simulink model "crazyflie_stu"  (R2021b)
settings: Solver=FixedStepDiscrete  StartTime=0.0  StopTime=160  FixedStep=0.001  RelTol=1e-3
undefined symbols (not defined in the file or in its folder): DiscIntNeverNeededParam
settings Model: PauseTimes=7  Creator=Zrean  LastModifiedBy=felix
settings SolverCC: AlgebraicLoopSolver=TrustRegion
settings DataIOCC: ReturnWorkspaceOutputs=off
settings OptimizationCC: DefaultParameterBehavior=Inlined  UseDivisionForNetSlopeComputation=on  UseFloatMulNetSlope=on  UseSpecifiedMinMax=on  InlineInvariantSignals=on  PassReuseOutputArgsAs=Individual arguments  ZeroExternalMemoryAtStartup=off  ZeroInternalMemoryAtStartup=off  NoFixptDivByZeroProtection=on  EfficientFloat2IntCast=on  LifeSpan=1  EfficientTunableParamExpr=on
settings DebuggingCC: AlgebraicLoopMsg=error  ParameterTunabilityLossMsg=error  SFMachineParentedDataDiag=warning  ArithmeticOperatorsInVariantConditions=warning
settings HardwareCC: ProdBitPerPointer=32  ProdBitPerSizeT=32  ProdBitPerPtrDiffT=32  ProdLargestAtomicInteger=Long  ProdLargestAtomicFloat=Double  ProdWordSize=32  ProdHWDeviceType=ARM Compatible->ARM Cortex
settings SFSimCC: SimUseLocalCustomCode=off  MATLABDynamicMemAlloc=off  CustomCodeUndefinedFunction=UseInterfaceOnly
settings RTWCC: Description=Embedded Coder  SystemTargetFile=ert.tlc  GenCodeOnly=on  TemplateMakefile=ert_default_tmf  GenerateReport=on  RTWUseLocalCustomCode=off  BuildConfiguration=Faster Runs  IncludeHyperlinkInReport=on  LaunchReport=on  GenerateTraceInfo=on  GenerateTraceReport=on  GenerateTraceReportSl=on  GenerateTraceReportSf=on  GenerateTraceReportEml=on  GenerateCodeMetricsReport=on
settings CodeAppCC: ForceParamTrailComments=on  IgnoreCustomStorageClasses=off  OperatorAnnotations=on  SimulinkDataObjDesc=on  SFDataObjDesc=on  MATLABFcnDesc=on  InsertBlockDesc=on  StateflowObjectComments=on  MATLABSourceComments=on
settings ERTTargetCC: TargetLangStandard=C99 (ISO)  MultiwordLength=2048  CombineSignalStateStructs=on  SuppressErrorStatus=on  SupportAbsoluteTime=off  SupportNonFinite=off  SupportComplex=off  InlinedParameterPlacement=NonHierarchical  ERTCustomFileTemplate=crazyflie_wrapper.tlc  ERTFilePackagingFormat=CompactWithDataFile
settings SimscapeCC: SimscapeNormalizeSystem=off

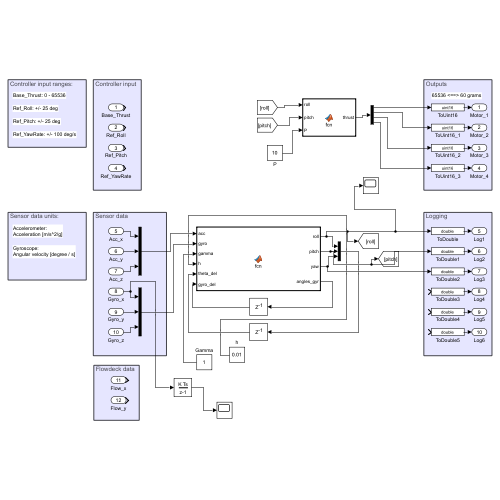
[thumbnail: Simulink's stored preview of the top-level diagram]
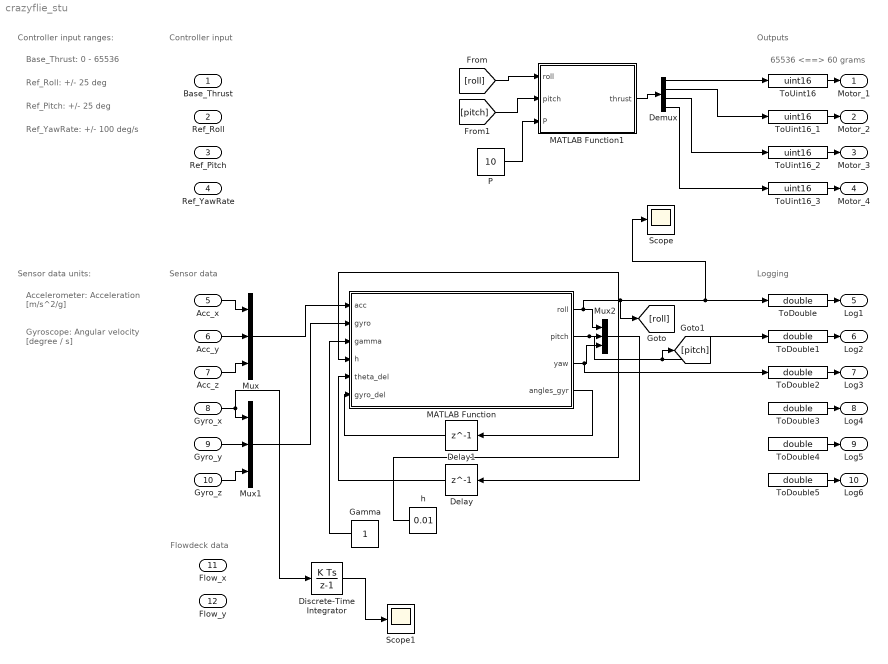
== system crazyflie_stu ==
  note: 65536 <==> 60 grams
  note: Logging
  note: Outputs
  note: Sensor data
  note: Controller input
  note: Ref_Roll: +/- 25 deg
  note: Base_Thrust: 0 - 65536
  note: Ref_Pitch: +/- 25 deg
  note: Ref_YawRate: +/- 100 deg/s
  note: Controller input ranges:
  note: Gyroscope:
      | Angular velocity [degree / s]
  note: Accelerometer:
      | Acceleration [m/s^2/g]
  note: Sensor data units:
  note: Flowdeck data
  Base_Thrust : Inport  OutDataTypeStr=double
  Ref_Roll : Inport  Port=2  OutDataTypeStr=double
  Ref_Pitch : Inport  Port=3  OutDataTypeStr=double
  Ref_YawRate : Inport  Port=4  OutDataTypeStr=double
  Acc_x : Inport  Port=5  OutDataTypeStr=double  PortDimensions=1
  Acc_y : Inport  Port=6  OutDataTypeStr=double  PortDimensions=1
  Acc_z : Inport  Port=7  OutDataTypeStr=double  PortDimensions=1
  Gyro_x : Inport  Port=8  OutDataTypeStr=double  PortDimensions=1
  Gyro_y : Inport  Port=9  OutDataTypeStr=double  PortDimensions=1
  Gyro_z : Inport  Port=10  OutDataTypeStr=double  PortDimensions=1
  Flow_x : Inport  Port=11  OutDataTypeStr=int16  PortDimensions=1
  Flow_y : Inport  Port=12  OutDataTypeStr=int16  PortDimensions=1
  Delay : Delay  DelayLength=1
  Delay1 : Delay  DelayLength=1
  Demux : Demux
  Discrete-Time Integrator : DiscreteIntegrator  SampleTime=-1  ICPrevOutput=DiscIntNeverNeededParam  ICPrevScaledInput=DiscIntNeverNeededParam
  Gamma : Constant
  MATLAB Function : MATLAB Function  TreatAsAtomicUnit=on
  MATLAB Function1 : MATLAB Function  TreatAsAtomicUnit=on
  Mux : Mux  Inputs=3
  Mux1 : Mux  Inputs=3
  Mux2 : Mux  Inputs=3
  P : Constant  Value=10
  Scope : Scope
  Scope1 : Scope
  ToDouble{,1..5} (6 alike) : DataTypeConversion  OutDataTypeStr=double  SaturateOnIntegerOverflow=on
  ToUint16 : DataTypeConversion  OutDataTypeStr=uint16  SaturateOnIntegerOverflow=on
  ToUint16_1 : DataTypeConversion  OutDataTypeStr=uint16  SaturateOnIntegerOverflow=on
  ToUint16_2 : DataTypeConversion  OutDataTypeStr=uint16  SaturateOnIntegerOverflow=on
  ToUint16_3 : DataTypeConversion  OutDataTypeStr=uint16  SaturateOnIntegerOverflow=on
  h : Constant  Value=0.01
  Motor_1 : Outport  OutDataTypeStr=uint16  VectorParamsAs1DForOutWhenUnconnected=off  LockScale=on
  Motor_2 : Outport  Port=2  OutDataTypeStr=uint16  VectorParamsAs1DForOutWhenUnconnected=off  LockScale=on
  Motor_3 : Outport  Port=3  OutDataTypeStr=uint16  VectorParamsAs1DForOutWhenUnconnected=off  LockScale=on
  Motor_4 : Outport  Port=4  OutDataTypeStr=uint16  VectorParamsAs1DForOutWhenUnconnected=off  LockScale=on
  Log1 : Outport  Port=5  OutDataTypeStr=double  VectorParamsAs1DForOutWhenUnconnected=off
  Log2 : Outport  Port=6  OutDataTypeStr=double  VectorParamsAs1DForOutWhenUnconnected=off
  Log3 : Outport  Port=7  OutDataTypeStr=double  VectorParamsAs1DForOutWhenUnconnected=off
  Log4 : Outport  Port=8  OutDataTypeStr=double  VectorParamsAs1DForOutWhenUnconnected=off
  Log5 : Outport  Port=9  OutDataTypeStr=double  VectorParamsAs1DForOutWhenUnconnected=off
  Log6 : Outport  Port=10  OutDataTypeStr=double  VectorParamsAs1DForOutWhenUnconnected=off
  wires:
  ToUint16/1 -> Motor_1/1
  ToUint16_1/1 -> Motor_2/1
  ToUint16_2/1 -> Motor_3/1
  ToUint16_3/1 -> Motor_4/1
  ToDouble/1 -> Log1/1
  ToDouble1/1 -> Log2/1
  ToDouble2/1 -> Log3/1
  ToDouble3/1 -> Log4/1
  ToDouble4/1 -> Log5/1
  ToDouble5/1 -> Log6/1
  Acc_x/1 -> Mux/1
  Acc_y/1 -> Mux/2
  Acc_z/1 -> Mux/3
  Gyro_x/1 -> Mux1/1, Discrete-Time Integrator/1
  Gyro_y/1 -> Mux1/2
  Gyro_z/1 -> Mux1/3
  Mux/1 -> MATLAB Function/1(acc)
  MATLAB Function/1(roll) -> Scope/1, ToDouble/1, [roll], Mux2/1
  MATLAB Function/2(pitch) -> [pitch], ToDouble1/1, Mux2/2
  Delay/1 -> MATLAB Function/5(theta_del)
  Mux2/1 -> Delay/1
  h/1 -> MATLAB Function/4(h)
  Gamma/1 -> MATLAB Function/3(gamma)
  MATLAB Function/4(angles_gyr) -> Delay1/1
  Delay1/1 -> MATLAB Function/6(gyro_del)
  MATLAB Function/3(yaw) -> ToDouble2/1, Mux2/3
  [roll] -> MATLAB Function1/1(roll)
  [pitch] -> MATLAB Function1/2(pitch)
  MATLAB Function1/1(thrust) -> Demux/1
  Demux/1 -> ToUint16/1
  Demux/2 -> ToUint16_1/1
  Demux/3 -> ToUint16_2/1
  Demux/4 -> ToUint16_3/1
  P/1 -> MATLAB Function1/3(P)
  Mux1/1 -> MATLAB Function/2(gyro)
  Discrete-Time Integrator/1 -> Scope1/1

== matlab function crazyflie_stu/MATLAB Function1 ==
  data: roll input; thrust output; pitch input; P input
function thrust = fcn(roll,pitch,P)


thrust = zeros(4,1);

roll_thrust = P*roll;
pitch_thrust = P*pitch;

thrust(1) =  roll_thrust + pitch_thrust;
thrust(2) =  roll_thrust - pitch_thrust;
thrust(3) = -roll_thrust - pitch_thrust;
thrust(4) = -roll_thrust + pitch_thrust;

thrust = min(65536,max(thrust,0));

== matlab function crazyflie_stu/MATLAB Function ==
  data: roll output size=1; acc input; pitch output size=1; yaw output size=1; gyro input; gamma input; h input; theta_del input; gyro_del input; angles_gyr output
function [roll, pitch, yaw, angles_gyr] = fcn(acc,gyro,gamma,h,theta_del,gyro_del)

%% Accelerometer to angles
phi_a = atan2d(-acc(2),-acc(3));
theta_a = atan2d(acc(1),sqrt(acc(2)^2+acc(3)^2));
angles_acc = [phi_a;theta_a; 0];

%% Gyro angles
phi_g = theta_del(1);
theta_g = theta_del(2);
psi_g = theta_del(3);

% 
% R_x = [1     0                0; 
%        0 cos(phi_g) -sin(phi_g); 
%        0 sin(phi_g)  cos(phi_g)];
% 
% R_y = [cos(theta_g)  0   sin(theta_g);
%        0             1              0;
%        -sin(theta_g) 0  cos(theta_g)];
% 
% R_z = [cos(psi_g) -sin(psi_g) 0;
%        sin(psi_g)  cos(psi_g) 0;
%        0            0         1];
% 
% w_R_b =R_x*R_y*R_z;
% b_R_w = R_x'*R_y'*R_z';


%angles_gyr = w_R_b*(gyro*h) + gyro_del;
angles_gyr = (gyro*h) + gyro_del;
%% Filter output
theta_k = (1-gamma)*angles_acc + gamma*(angles_gyr);

disp(h)
disp(gamma)

roll = theta_k(1);
pitch = theta_k(2);
yaw = theta_k(3);
